simulink model "Tarea_Bloques"  (R2021b)
settings: Solver=VariableStepAuto  StartTime=0.0  StopTime=10.0  RelTol=1e-3
undefined symbols (not defined in the file or in its folder): G1, G2, G3, G4, H1
libraries: cstblocks x6
settings Model: Creator=Duván Ramírez Lotta  LastModifiedBy=Duván Ramírez Lotta

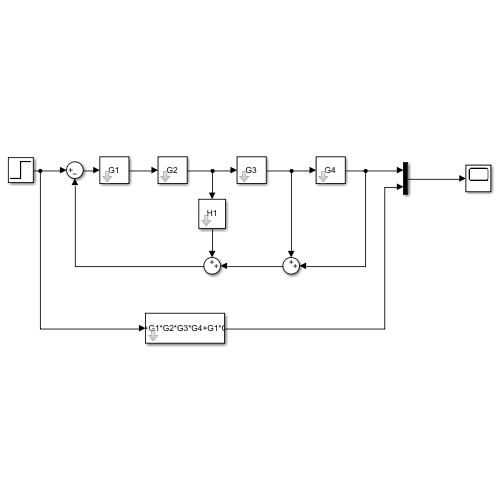
[thumbnail: Simulink's stored preview of the top-level diagram]
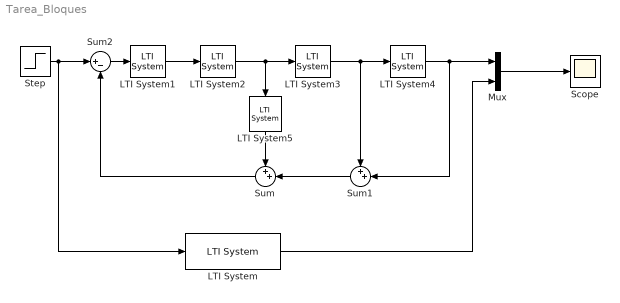
== system Tarea_Bloques ==
  LTI System : cstblocks/LTI System  sys=[G1*G2*G3*G4]/[1+G1*G2*G3*G4+G1*G2*H1+G1*G2*G3]  IC=[]
  LTI System1 : cstblocks/LTI System  sys=G1  IC=[]
  LTI System2 : cstblocks/LTI System  sys=G2  IC=[]
  LTI System3 : cstblocks/LTI System  sys=G3  IC=[]
  LTI System4 : cstblocks/LTI System  sys=G4  IC=[]
  LTI System5 : cstblocks/LTI System  sys=H1  IC=[]
  Mux : Mux  Inputs=2
  Scope : Scope
  Step : Step  SampleTime=0
  Sum : Sum  Inputs=++|
  Sum1 : Sum  Inputs=++|
  Sum2 : Sum  Inputs=|+-
  wires:
  Mux/1 -> Scope/1
  Sum1/1 -> Sum/2
  Step/1 -> LTI System/1, Sum2/1
  Sum2/1 -> LTI System1/1
  LTI System1/1 -> LTI System2/1
  LTI System2/1 -> LTI System5/1, LTI System3/1
  LTI System3/1 -> Sum1/1, LTI System4/1
  LTI System4/1 -> Sum1/2, Mux/1
  LTI System5/1 -> Sum/1
  Sum/1 -> Sum2/2
  LTI System/1 -> Mux/2
